simulink model "modelo_simulink"  (R2021a)
settings: Solver=VariableStepAuto  StartTime=0.0  StopTime=100  RelTol=1e-3
libraries: simulink x1
settings Model: Creator=phcs  LastModifiedBy=phcs

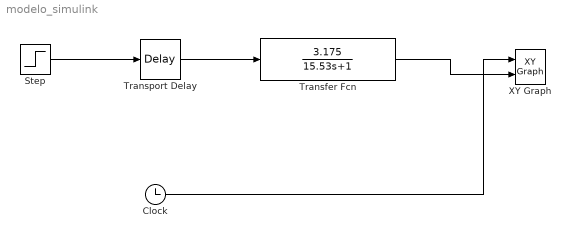
== system modelo_simulink ==
  Clock : Clock
  Step : Step  Time=0  After=0.4  SampleTime=0
  Transfer Fcn : TransferFcn  Numerator=[3.175]  Denominator=[15.53 1]
  Transport Delay : TransportDelay  DelayTime=2.88
  XY Graph : simulink/Sinks/XY Graph  xmin=0  xmax=100  ymin=-0  ymax=1.5  st=0
  wires:
  Step/1 -> Transport Delay/1
  Transport Delay/1 -> Transfer Fcn/1
  Transfer Fcn/1 -> XY Graph/2
  Clock/1 -> XY Graph/1
